simulink model "AACBlocks"  (R2019b)
settings: Solver=VariableStepAuto  StartTime=0.0  StopTime=100  RelTol=1e-3
libraries: cstblocks x3, simulink x1
settings Model: Creator=daose  LastModifiedBy=daose
settings SolverCC: AlgebraicLoopSolver=LineSearch
settings DebuggingCC: AlgebraicLoopMsg=none

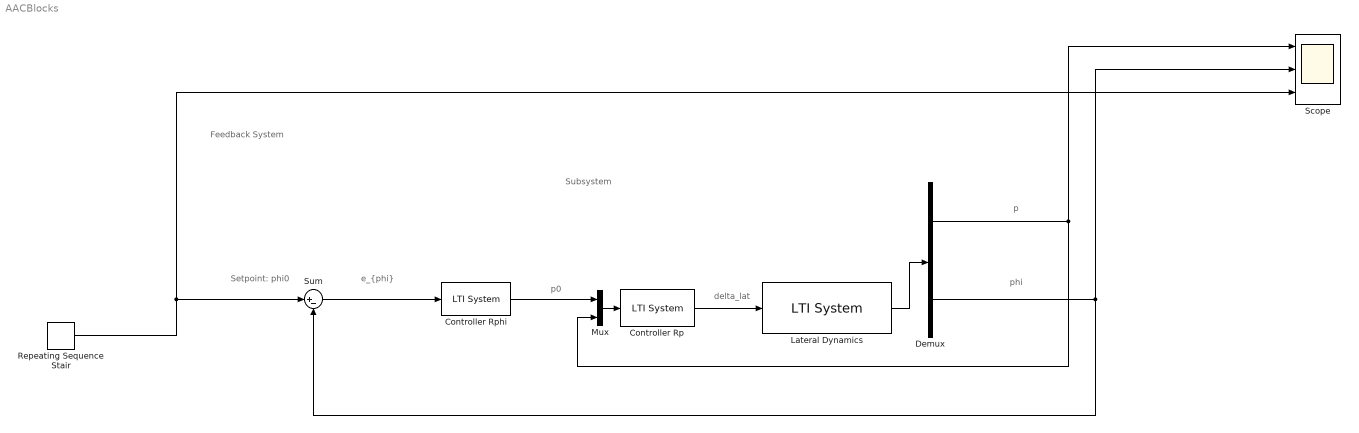
== system AACBlocks ==
  note: Feedback System
  note: phi
  note: p
  note: delta_lat
  note: p0
  note: Setpoint: phi0
  note: e_{phi}
  note: Subsystem
  Controller Rp : cstblocks/LTI System  sys=Rp  IC=[]
  Controller Rphi : cstblocks/LTI System  sys=Rphi  IC=[]
  Demux : Demux  Outputs=2
  Lateral Dynamics : cstblocks/LTI System  sys=G  IC=[]
  Mux : Mux  Inputs=2
  Repeating Sequence Stair : simulink/Sources/Repeating Sequence Stair  OutValues=[3 1 4 2 1].'  tsamp=10  OutMin=[]  OutMax=[]  OutDataTypeStr=double  OutputDataTypeScalingMode=double  OutDataType=fixdt(0,8)  ConRadixGroup=Best Precision: Vector-wise  OutScaling=2^-12
  Scope : Scope  NumInputPorts=3
  Sum : Sum  Inputs=|+-
  wires:
  Controller Rp/1 -> Lateral Dynamics/1
  Mux/1 -> Controller Rp/1
  Lateral Dynamics/1 -> Demux/1
  Controller Rphi/1 -> Mux/1
  Sum/1 -> Controller Rphi/1
  Repeating Sequence Stair/1 -> Scope/3, Sum/1
  Demux/2 -> Sum/2, Scope/2
  Demux/1 -> Mux/2, Scope/1
